simulink model "Simulation_3DOF02Testing01"  (R2024a)
settings: Solver=ode4  StartTime=initial_time  StopTime=final_time  FixedStep=timestep  RelTol=1e-3
values from neighbouring files (symbols this model uses):
  alphaArray = [-30, -25, -20, -15, -10, -5, 0, 5, 10, 15, 20, 25, 30]    [Constants_3DOF.m]
  altitudeArray = [0, 1000, 2000, 3000, 4000, 5000, 6000, 7000, 8000, 9000, 10000, 15000, 20000,      25000, 30000, 35000, 40000, 45000, 50000, 55000, 60000]    [Constants_3DOF.m]
  cD_3DArray = zeros(numAoAs, numMachs, numAltitudes)    [Constants_3DOF.m]
  cL_3DArray = zeros(numAoAs, numMachs, numAltitudes)    [Constants_3DOF.m]
  flight_path_angle_0 = flight_path_angle_0 * (pi / 180)    (= 0.0523598775598)    [Constants_3DOF.m]
  heading_angle_0 = heading_angle_0 * (pi/180)    (= 0.349065850399)    [Constants_3DOF.m]
  height_0 = 35 * 10^3    (= 35000)    [Constants_3DOF.m]
  heightsList = usAtmosphere.Z    [Constants_3DOF.m]
  latitude_0 = latitude_0 * (pi/180)    (= 0.680503875353)    [Constants_3DOF.m]
  longitude_0 = longitude_0 * (pi/180)    (= -1.26396744429)    [Constants_3DOF.m]
  machArray = [0.5, 1.0, 1.5, 2.0, 2.5, 3.0, 3.5, 4.0, 4.5, 5.0, 5.5, 6.0, 6.5, 7.0, 7.5, 8.0,      8.5, 9.0, 9.5, 10.0]    [Constants_3DOF.m]
  mass = 161.5    [Constants_3DOF.m]
  omega_earth = 7.2921159 * 10^-5    (= 7.2921159e-05)    [Constants_3DOF.m]
  optimalAoA = zeros(numMachs, numAltitudes)    [Constants_3DOF.m]
  r_earth = 6371.0088 * 10^3    (= 6371008.8)    [Constants_3DOF.m]
  range_0 = 0    [Constants_3DOF.m]
  range_to_go_0 = 11112 * 10^3    (= 11112000)    [Constants_3DOF.m]
  rhoList = usAtmosphere.x_    [Constants_3DOF.m]
  speed_0 = 1500    [Constants_3DOF.m]
  temperatureList = usAtmosphere.T    [Constants_3DOF.m]
  wing_area = 0.079813    [Constants_3DOF.m]
libraries: simulink_extras x5
settings Model: Creator=641893  LastModifiedBy=641893

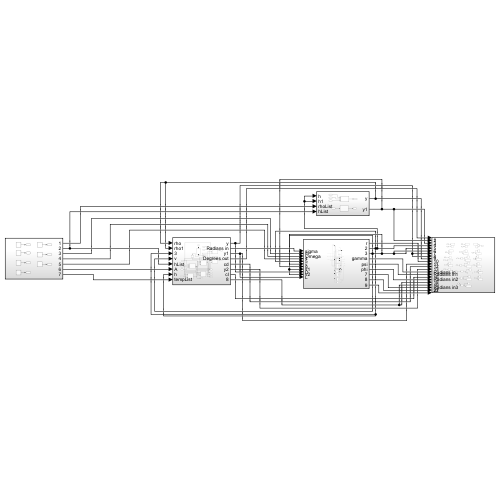
[thumbnail: Simulink's stored preview of the top-level diagram]
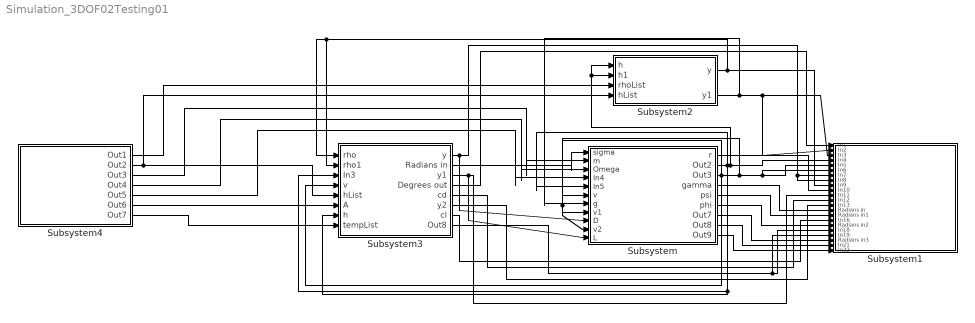
== system Simulation_3DOF02Testing01 ==
  Subsystem : Subsystem
  Subsystem1 : Subsystem
  Subsystem2 : Subsystem
  Subsystem3 : Subsystem
  Subsystem4 : Subsystem
  wires:
  Subsystem/2(Out2) -> Subsystem3/3(In3), Subsystem3/7(h), Subsystem2/2(h1), Subsystem2/1(h), Subsystem1/4(In4), Subsystem/5(In5)
  Subsystem/3(Out3) -> Subsystem1/5(In5), Subsystem1/6(In6), Subsystem/6(v), Subsystem/8(v1), Subsystem/10(v2), Subsystem3/4(v)
  Subsystem/1(r) -> Subsystem1/10(In10)
  Subsystem/4(gamma) -> Subsystem1/14(Radians in)
  Subsystem/5(psi) -> Subsystem1/15(Radians in1)
  Subsystem/6(phi) -> Subsystem1/17(Radians in2)
  Subsystem/7(Out7) -> Subsystem1/20(Radians in3)
  Subsystem/8(Out8) -> Subsystem1/21(In21)
  Subsystem/9(Out9) -> Subsystem1/22(In22)
  Subsystem2/2(y1) -> Subsystem1/3(In3), Subsystem1/2(In2), Subsystem/7(g)
  Subsystem2/1(y) -> Subsystem3/2(rho1), Subsystem3/1(rho), Subsystem1/9(In9)
  Subsystem3/1(y) -> Subsystem1/7(In7), Subsystem1/8(In8), Subsystem/9(D)
  Subsystem3/3(y1) -> Subsystem/11(L), Subsystem1/11(In11)
  Subsystem3/8(Out8) -> Subsystem1/19(In19), Subsystem1/18(In18)
  Subsystem3/2(Radians in) -> Subsystem/1(sigma)
  Subsystem3/4(Degrees out) -> Subsystem1/1(In1)
  Subsystem3/5(cd) -> Subsystem1/12(In12)
  Subsystem3/6(y2) -> Subsystem1/13(In13)
  Subsystem3/7(cl) -> Subsystem1/16(In16)
  Subsystem4/2(Out2) -> Subsystem3/5(hList), Subsystem2/4(hList)
  Subsystem4/1(Out1) -> Subsystem2/3(rhoList)
  Subsystem4/3(Out3) -> Subsystem/2(m)
  Subsystem4/4(Out4) -> Subsystem/3(Omega)
  Subsystem4/5(Out5) -> Subsystem/4(In4)
  Subsystem4/6(Out6) -> Subsystem3/6(A)
  Subsystem4/7(Out7) -> Subsystem3/8(tempList)

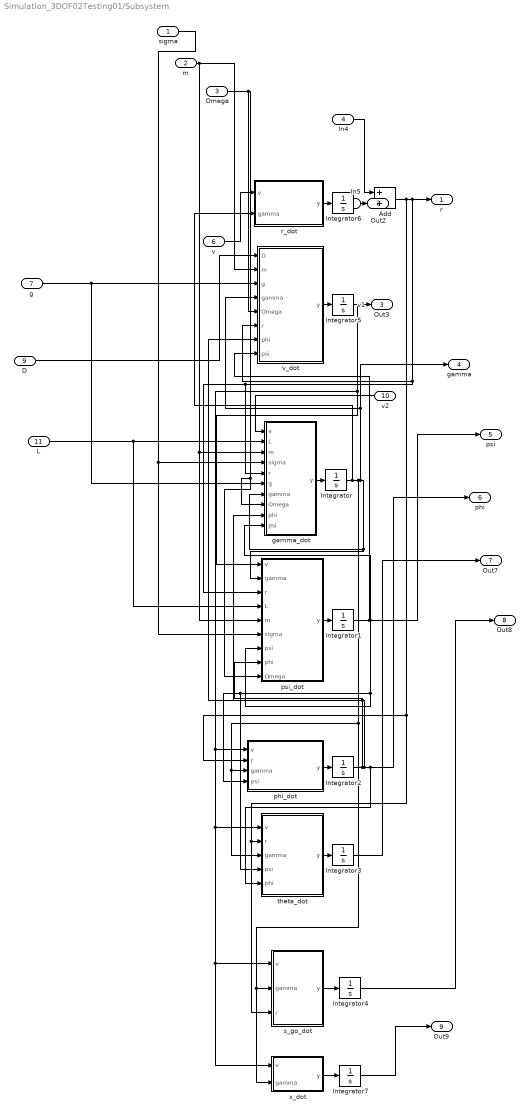
== system Simulation_3DOF02Testing01/Subsystem ==
  sigma : Inport
  m : Inport  Port=2
  Omega : Inport  Port=3
  In4 : Inport  Port=4
  In5 : Inport  Port=5
  v : Inport  Port=6
  g : Inport  Port=7
  v1 : Inport  Port=8
  D : Inport  Port=9
  v2 : Inport  Port=10
  L : Inport  Port=11
  " x_dot" : MATLAB Function  TreatAsAtomicUnit=on
  Add : Sum
  Integrator : Integrator  InitialCondition=flight_path_angle_0
  Integrator1 : Integrator  InitialCondition=heading_angle_0
  Integrator2 : Integrator  InitialCondition=latitude_0
  Integrator3 : Integrator  InitialCondition=longitude_0
  Integrator4 : Integrator  InitialCondition=range_to_go_0
  Integrator5 : Integrator  InitialCondition=speed_0
  Integrator6 : Integrator  InitialCondition=height_0
  Integrator7 : Integrator  InitialCondition=range_0
  gamma_dot : MATLAB Function  TreatAsAtomicUnit=on
  phi_dot : MATLAB Function  TreatAsAtomicUnit=on
  psi_dot : MATLAB Function  TreatAsAtomicUnit=on
  r_dot : MATLAB Function  TreatAsAtomicUnit=on
  s_go_dot : MATLAB Function  TreatAsAtomicUnit=on
  theta_dot : MATLAB Function  TreatAsAtomicUnit=on
  v_dot : MATLAB Function  TreatAsAtomicUnit=on
  r : Outport
  Out2 : Outport  Port=2
  Out3 : Outport  Port=3
  gamma : Outport  Port=4
  psi : Outport  Port=5
  phi : Outport  Port=6
  Out7 : Outport  Port=7
  Out8 : Outport  Port=8
  Out9 : Outport  Port=9
  wires:
  Integrator1/1 -> phi_dot/4(psi), theta_dot/4(psi), psi_dot/7(psi), gamma_dot/10(psi), psi/1, v_dot/8(psi)
  " x_dot"/1(y) -> Integrator7/1
  Integrator2/1 -> phi/1, theta_dot/5(phi), v_dot/7(phi), gamma_dot/9(phi), psi_dot/8(phi)
  gamma_dot/1(y) -> Integrator/1
  sigma/1 -> psi_dot/6(sigma), gamma_dot/4(sigma)
  In5/1 -> Add/2
  v_dot/1(y) -> Integrator5/1
  r_dot/1(y) -> Integrator6/1
  v1/1 -> s_go_dot/1(v), " x_dot"/1(v), theta_dot/1(v), phi_dot/1(v), psi_dot/1(v)
  Add/1 -> theta_dot/2(r), s_go_dot/3(r), phi_dot/2(r), gamma_dot/5(r), psi_dot/3(r), v_dot/6(r), r/1
  psi_dot/1(y) -> Integrator1/1
  Integrator5/1 -> Out3/1
  s_go_dot/1(y) -> Integrator4/1
  theta_dot/1(y) -> Integrator3/1
  phi_dot/1(y) -> Integrator2/1
  Integrator/1 -> s_go_dot/2(gamma), " x_dot"/2(gamma), theta_dot/3(gamma), phi_dot/3(gamma), psi_dot/2(gamma), gamma_dot/7(gamma), gamma/1, v_dot/4(gamma), r_dot/2(gamma)
  Integrator6/1 -> Out2/1
  Omega/1 -> gamma_dot/8(Omega), psi_dot/9(Omega), v_dot/5(Omega)
  m/1 -> gamma_dot/3(m), psi_dot/5(m), v_dot/2(m)
  g/1 -> gamma_dot/6(g), v_dot/3(g)
  In4/1 -> Add/1
  L/1 -> gamma_dot/2(L), psi_dot/4(L)
  v2/1 -> gamma_dot/1(v)
  v/1 -> r_dot/1(v)
  Integrator3/1 -> Out7/1
  Integrator4/1 -> Out8/1
  Integrator7/1 -> Out9/1
  D/1 -> v_dot/1(D)

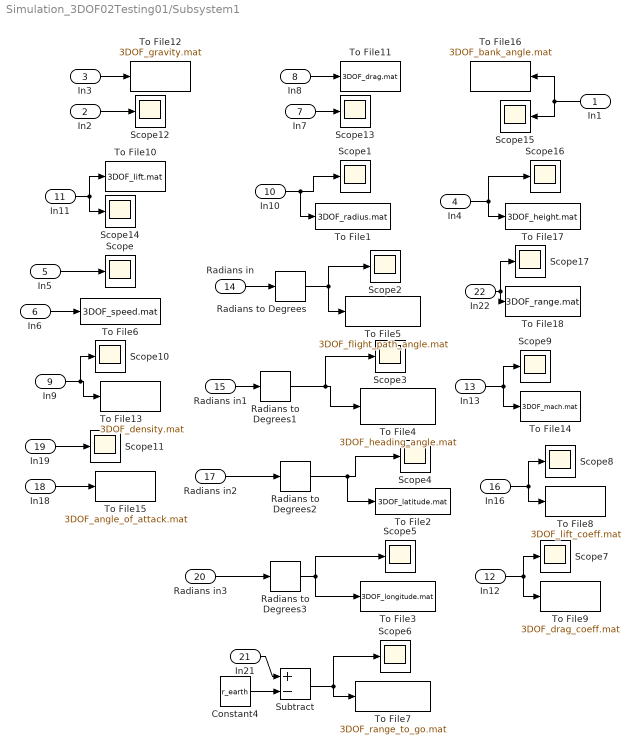
== system Simulation_3DOF02Testing01/Subsystem1 ==
  In1 : Inport
  In2 : Inport  Port=2
  In3 : Inport  Port=3
  In4 : Inport  Port=4
  In5 : Inport  Port=5
  In6 : Inport  Port=6
  In7 : Inport  Port=7
  In8 : Inport  Port=8
  In9 : Inport  Port=9
  In10 : Inport  Port=10
  In11 : Inport  Port=11
  In12 : Inport  Port=12
  In13 : Inport  Port=13
  Radians in : Inport  Port=14
  Radians in1 : Inport  Port=15
  In16 : Inport  Port=16
  Radians in2 : Inport  Port=17
  In18 : Inport  Port=18
  In19 : Inport  Port=19
  Radians in3 : Inport  Port=20
  In21 : Inport  Port=21
  In22 : Inport  Port=22
  Constant4 : Constant  Value=r_earth
  Radians to Degrees{,1..3} (4 alike) : simulink_extras/Transformations/Radians to Degrees
  Scope{,1..17} (18 alike) : Scope
  Subtract : Sum  Inputs=+-
  To File1 : ToFile  Filename=3DOF_radius.mat
  To File10 : ToFile  Filename=3DOF_lift.mat
  To File11 : ToFile  Filename=3DOF_drag.mat
  To File12 : ToFile  Filename=3DOF_gravity.mat
  To File13 : ToFile  Filename=3DOF_density.mat
  To File14 : ToFile  Filename=3DOF_mach.mat
  To File15 : ToFile  Filename=3DOF_angle_of_attack.mat
  To File16 : ToFile  Filename=3DOF_bank_angle.mat
  To File17 : ToFile  Filename=3DOF_height.mat
  To File18 : ToFile  Filename=3DOF_range.mat
  To File2 : ToFile  Filename=3DOF_latitude.mat
  To File3 : ToFile  Filename=3DOF_longitude.mat
  To File4 : ToFile  Filename=3DOF_heading_angle.mat
  To File5 : ToFile  Filename=3DOF_flight_path_angle.mat
  To File6 : ToFile  Filename=3DOF_speed.mat
  To File7 : ToFile  Filename=3DOF_range_to_go.mat
  To File8 : ToFile  Filename=3DOF_lift_coeff.mat
  To File9 : ToFile  Filename=3DOF_drag_coeff.mat
  wires:
  In10/1 -> Scope1/1, To File1/1
  Radians to Degrees1/1 -> To File4/1, Scope3/1
  In13/1 -> To File14/1, Scope9/1
  Radians in1/1 -> Radians to Degrees1/1
  In7/1 -> Scope13/1
  In4/1 -> To File17/1, Scope16/1
  Subtract/1 -> Scope6/1, To File7/1
  Radians to Degrees2/1 -> To File2/1, Scope4/1
  Radians in/1 -> Radians to Degrees/1
  Radians in2/1 -> Radians to Degrees2/1
  In1/1 -> To File16/1, Scope15/1
  Radians to Degrees3/1 -> To File3/1, Scope5/1
  In11/1 -> Scope14/1, To File10/1
  In16/1 -> To File8/1, Scope8/1
  In9/1 -> To File13/1, Scope10/1
  In21/1 -> Subtract/1
  In22/1 -> Scope17/1, To File18/1
  Radians to Degrees/1 -> Scope2/1, To File5/1
  In3/1 -> To File12/1
  In2/1 -> Scope12/1
  In12/1 -> To File9/1, Scope7/1
  Constant4/1 -> Subtract/2
  In19/1 -> Scope11/1
  In5/1 -> Scope/1
  In6/1 -> To File6/1
  In8/1 -> To File11/1
  In18/1 -> To File15/1
  Radians in3/1 -> Radians to Degrees3/1

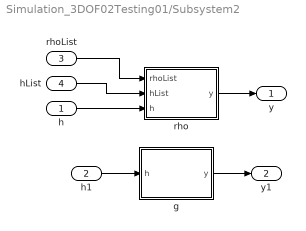
== system Simulation_3DOF02Testing01/Subsystem2 ==
  h : Inport
  h1 : Inport  Port=2
  rhoList : Inport  Port=3
  hList : Inport  Port=4
  g : MATLAB Function  TreatAsAtomicUnit=on
  rho : MATLAB Function  TreatAsAtomicUnit=on
  y : Outport
  y1 : Outport  Port=2
  wires:
  h/1 -> rho/3(h)
  rhoList/1 -> rho/1(rhoList)
  g/1(y) -> y1/1
  rho/1(y) -> y/1
  hList/1 -> rho/2(hList)
  h1/1 -> g/1(h)

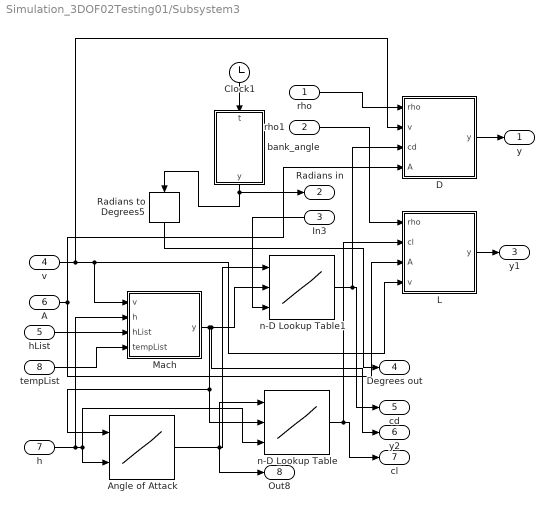
== system Simulation_3DOF02Testing01/Subsystem3 ==
  rho : Inport
  rho1 : Inport  Port=2
  In3 : Inport  Port=3
  v : Inport  Port=4
  hList : Inport  Port=5
  A : Inport  Port=6
  h : Inport  Port=7
  tempList : Inport  Port=8
  Angle of Attack : Lookup_n-D  BreakpointsForDimension1=machArray  BreakpointsForDimension2=altitudeArray  BreakpointsForDimension3=altitudeArray  Table=optimalAoA  InterpMethod=Linear Lagrange  InternalRulePriority=Speed  RndMeth=Simplest
      settings: InputPortMap=u0,u1
  Clock1 : Clock
  D : MATLAB Function  TreatAsAtomicUnit=on
  L : MATLAB Function  TreatAsAtomicUnit=on
  Mach : MATLAB Function  TreatAsAtomicUnit=on
  Radians to Degrees5 : simulink_extras/Transformations/Radians to Degrees
  bank_angle : MATLAB Function  TreatAsAtomicUnit=on
  n-D Lookup Table : Lookup_n-D  NumberOfTableDimensions=3  BreakpointsForDimension1=alphaArray  BreakpointsForDimension2=machArray  BreakpointsForDimension3=altitudeArray  IndexSearchMethod=Linear search  Table=cL_3DArray  InterpMethod=Linear Lagrange  InternalRulePriority=Speed  RndMeth=Simplest
      settings: InputPortMap=u0,u1,u2
  n-D Lookup Table1 : Lookup_n-D  NumberOfTableDimensions=3  BreakpointsForDimension1=alphaArray  BreakpointsForDimension2=machArray  BreakpointsForDimension3=altitudeArray  IndexSearchMethod=Linear search  Table=cD_3DArray  InterpMethod=Linear Lagrange  InternalRulePriority=Speed  RndMeth=Simplest
      settings: InputPortMap=u0,u1,u2
  y : Outport
  Radians in : Outport  Port=2
  y1 : Outport  Port=3
  Degrees out : Outport  Port=4
  cd : Outport  Port=5
  y2 : Outport  Port=6
  cl : Outport  Port=7
  Out8 : Outport  Port=8
  wires:
  Clock1/1 -> bank_angle/1(t)
  v/1 -> L/4(v), Mach/1(v), D/2(v)
  A/1 -> D/4(A), L/3(A)
  rho/1 -> D/1(rho)
  bank_angle/1(y) -> Radians in/1, Radians to Degrees5/1
  n-D Lookup Table1/1 -> D/3(cd), cd/1
  h/1 -> Angle of Attack/2, n-D Lookup Table/3, Mach/2(h)
  Mach/1(y) -> n-D Lookup Table/2, Angle of Attack/1, y2/1, n-D Lookup Table1/2
  Angle of Attack/1 -> Out8/1, n-D Lookup Table1/1, n-D Lookup Table/1
  Radians to Degrees5/1 -> Degrees out/1
  n-D Lookup Table/1 -> L/2(cl), cl/1
  hList/1 -> Mach/3(hList)
  tempList/1 -> Mach/4(tempList)
  D/1(y) -> y/1
  In3/1 -> n-D Lookup Table1/3
  rho1/1 -> L/1(rho)
  L/1(y) -> y1/1

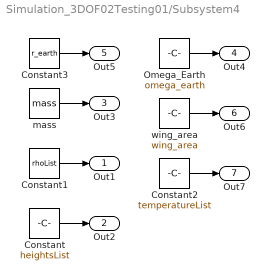
== system Simulation_3DOF02Testing01/Subsystem4 ==
  Constant : Constant  Value=heightsList
  Constant1 : Constant  Value=rhoList
  Constant2 : Constant  Value=temperatureList
  Constant3 : Constant  Value=r_earth
  Omega_Earth : Constant  Value=omega_earth
  mass : Constant  Value=mass
  wing_area : Constant  Value=wing_area
  Out1 : Outport
  Out2 : Outport  Port=2
  Out3 : Outport  Port=3
  Out4 : Outport  Port=4
  Out5 : Outport  Port=5
  Out6 : Outport  Port=6
  Out7 : Outport  Port=7
  wires:
  Omega_Earth/1 -> Out4/1
  wing_area/1 -> Out6/1
  Constant/1 -> Out2/1
  Constant1/1 -> Out1/1
  Constant3/1 -> Out5/1
  Constant2/1 -> Out7/1
  mass/1 -> Out3/1

== matlab function Simulation_3DOF02Testing01/Subsystem3/D ==
  data: rho input; y output; v input; cd input; A input
function y = fcn(rho, v, cd, A)

y = 0.5 * rho * v^2 * A * cd;

== matlab function Simulation_3DOF02Testing01/Subsystem2/g ==
  data: y output; h input
function y = fcn(h)
mu_earth = 3.96272 * 10^14;
rE = 6378140;
y = mu_earth / (rE + h)^2;

== matlab function Simulation_3DOF02Testing01/Subsystem2/rho ==
  data: rhoList input; hList input; h input; y output
function y = fcn(rhoList, hList,h)

h = h / 10^3;

if h >= 0
    density = interp1(hList, rhoList, h);
else
    density = 0;
end


y = density;

== matlab function Simulation_3DOF02Testing01/Subsystem/ x_dot ==
  data: v input; y output; gamma input
function y = fcn(v, gamma)

y = v * cos(gamma);

== matlab function Simulation_3DOF02Testing01/Subsystem3/Mach ==
  data: v input; y output; h input; hList input; tempList input
function y = fcn(v, h, hList, tempList)

gamma = 1.4;
R = 287.05;

h = h / 10^3;

if h >= 0
    temp = interp1(hList, tempList, h);
    a = sqrt(gamma * R * temp);
    y = v/a;
else
    temp = 0;
    y = 0;
end

== matlab function Simulation_3DOF02Testing01/Subsystem3/bank_angle ==
  data: t input; y output
function y = fcn(t)

sigma = 0;
sigma = sigma * pi / 180;

y = sigma;

== matlab function Simulation_3DOF02Testing01/Subsystem/phi_dot ==
  data: v input; y output; r input; gamma input; psi input
function y = fcn(v, r, gamma, psi)

y = (v / r) * cos(gamma) * sin(psi);

== matlab function Simulation_3DOF02Testing01/Subsystem/r_dot ==
  data: v input; y output; gamma input
function y = fcn(v, gamma)

y = v * sin(gamma);

== matlab function Simulation_3DOF02Testing01/Subsystem/theta_dot ==
  data: v input; y output; r input; gamma input; psi input; phi input
function y = fcn(v, r, gamma, psi, phi)

y = (v * cos(gamma) * cos(psi) ) / (r * cos(phi) );

== matlab function Simulation_3DOF02Testing01/Subsystem/v_dot ==
  data: D input; y output; m input; g input; gamma input; Omega input; r input; phi input; psi input
function y = fcn(D, m, g, gamma, Omega, r, phi, psi)

y = -(D / m) - g * sin(gamma) + Omega^2 * r * cos(phi) * ( sin(gamma) * cos(phi) - cos(gamma) * sin(phi) * cos(psi) );

== matlab function Simulation_3DOF02Testing01/Subsystem/gamma_dot ==
  data: v input; y output; L input; m input; sigma input; r input; g input; gamma input; Omega input; phi input; psi input
function y = fcn(v, L, m, sigma, r, g, gamma, Omega, phi, psi)

y = (1/v) * ( (L / m) * cos(sigma) + (( v^2 / r) - g) * cos(gamma) + 2 * Omega * v * cos(phi) * sin(psi) + Omega^2 * r * cos(phi) * ( cos(gamma) * cos(phi) - sin(gamma) * sin(phi) * cos(psi) ) );

== matlab function Simulation_3DOF02Testing01/Subsystem/psi_dot ==
  data: v input; y output; gamma input; r input; L input; m input; sigma input; psi input; phi input; Omega input
function y = fcn(v, gamma, r, L, m, sigma, psi, phi, Omega)

y = (1 / v) * ( (L / (m * cos(gamma))) * sin(sigma) + (v^2 /  r) * cos(gamma) * sin(psi) * tan(phi) - 2 * Omega * v * (tan(gamma) * cos(psi) * cos(phi) - sin(phi) ) + (Omega^2 * r / cos(gamma)) * sin(psi) * sin(phi) * cos(phi) );

== matlab function Simulation_3DOF02Testing01/Subsystem/s_go_dot ==
  data: v input; y output; gamma input; r input
function y = fcn(v, gamma, r)
rE = 6378140;
y = -v * cos(gamma) * rE / r;

== matlab function Simulation_3DOF02Testing01/Subsystem3/L ==
  data: rho input; y output; cl input; A input; v input
function y = fcn(rho, cl, A, v)

y = 0.5 * rho * v^2 * A * cl;
